simulink model "OpenLoop"  (R2022b)
settings: Solver=ode1  StartTime=0.0  StopTime=10  FixedStep=0.002  RelTol=1e-3  EnableMultiTasking=on
undefined symbols (not defined in the file or in its folder): sigbuilder_block
libraries: simulink x1
settings Model: SimulationMode=external  ExtModeTrigDuration=2  Creator=Alex  LastModifiedBy=lgoudal
settings SolverCC: AlgebraicLoopSolver=TrustRegion
settings DataIOCC: SaveFormat=StructureWithTime  ReturnWorkspaceOutputs=off
settings OptimizationCC: PassReuseOutputArgsAs=Individual arguments  MaxStackSize=64  EfficientTunableParamExpr=on
settings DebuggingCC: ParameterTunabilityLossMsg=error  UnconnectedInputMsg=warning  UnconnectedOutputMsg=warning  UnconnectedLineMsg=warning  SFMachineParentedDataDiag=warning  ArithmeticOperatorsInVariantConditions=warning
settings HardwareCC: ProdBitPerInt=16  ProdBitPerPointer=16  ProdBitPerSizeT=16  ProdBitPerPtrDiffT=16  ProdLargestAtomicFloat=None  ProdWordSize=8  ProdHWDeviceType=Atmel->AVR
settings ModelReferenceCC: EnableRefExpFcnMdlSchedulingChecks=on
settings SFSimCC: SimUseLocalCustomCode=off  MATLABDynamicMemAlloc=off  CustomCodeUndefinedFunction=UseInterfaceOnly
settings RTWCC: Description=Embedded Coder  SystemTargetFile=ert.tlc  HardwareBoard=Arduino Mega 2560  TemplateMakefile=ert_default_tmf  RTWUseLocalCustomCode=off  Toolchain=Arduino AVR  BuildConfiguration=Faster Runs  IncludeHyperlinkInReport=on  DLArmComputeVersion=19.05
settings CodeAppCC: ForceParamTrailComments=on  IgnoreCustomStorageClasses=off  OperatorAnnotations=on  SimulinkDataObjDesc=on  SFDataObjDesc=on  InsertBlockDesc=on
settings ERTTargetCC: SupportContinuousTime=on  SupportVariableSizeSignals=on  ExtMode=on  ExtModeTransport=3  ExtModeStaticAlloc=on  ExtModeMexFile=ext_xcp  ExtModeMexArgs=0 10 115200  ExtModeIntrfLevel=Level2 - Open

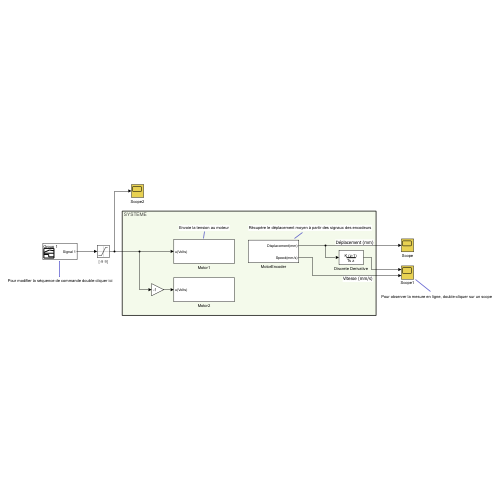
[thumbnail: Simulink's stored preview of the top-level diagram]
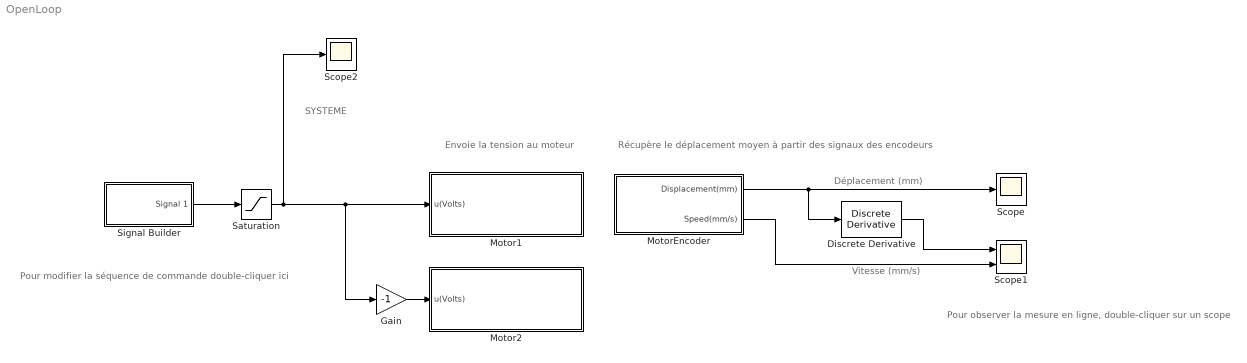
== system OpenLoop ==
  note: Déplacement (mm)
  note: Vitesse (mm/s)
  note: SYSTEME
  note: Récupère le déplacement moyen à partir des signaux des encodeurs
  note: Envoie la tension au moteur
  note: Pour observer la mesure en ligne, double-cliquer sur un scope
  note: Pour modifier la séquence de commande double-cliquer ici
  Discrete Derivative : simulink/Discrete/Discrete Derivative  gainval=1.0  ICPrevScaledInput=0.0  OutMin=[]  OutMax=[]  OutDataType=fixdt(1, 16)  OutScaling=2^-10  DoSatur=off
  Gain : Gain  Gain=-1
  Motor1 : Subsystem  mask{Vmax=12}
      mask prompts: Vmax "Power supply Voltage"
  Motor2 : Subsystem  mask{Vmax=12}
      mask prompts: Vmax "Power supply Voltage"
  MotorEncoder : Subsystem  mask{pulsePerTurn=8, beltPitch=2.032, nTeeth=90, gearRatio=46}
      mask prompts: pulsePerTurn "Encoder resolution"; beltPitch "Belt Pitch"; nTeeth "Number of teeth"; gearRatio "Gear ratio"
  Saturation : Saturate  UpperLimit=9  LowerLimit=-9
      settings: AttributesFormatString=[%<LowerLimit> %<UpperLimit>]
  Scope : Scope
  Scope1 : Scope  NumInputPorts=2
  Scope2 : Scope
  Signal Builder : Subsystem  Tag=STV Subsys  LoadFcn=sigbuilder_block('load');  StartFcn=sigbuilder_block('start');  StopFcn=sigbuilder_block('stop');  ClipboardFcn=sigbuilder_block('clipboard');  mask(Sigbuilder block){tuvar=[0:10]}
      mask help: Simulink:masks:SigbuilderBlock_MD
      mask init:
      | if ~strcmp(get_param(bdroot(gcbh),'SimulationStatus'),'stopped') tuvar = sigbuilder_block('maskInit'); end
      settings: CopyFcn=sigbuilder_block('copy');  DeleteFcn=sigbuilder_block('delete');  ModelCloseFcn=sigbuilder_block('modelClose');  PreSaveFcn=sigbuilder_block('preSave');  PauseFcn=sigbuilder_block('pause');  ContinueFcn=sigbuilder_block('continue');  NameChangeFcn=sigbuilder_block('namechange');  OpenFcn=sigbuilder_block('open',[382.125 217.125 550.5 400.5 ]);  CloseFcn=sigbuilder_block('close');
      mask Display: plot(0, 0, 100, 100,[2, 2, 32, 32, 2], [68, 8, 8, 68, 68],[32, 2], [38, 38], [32, 19, 2],[53, 60, 44], [32, 17, 17, 2],[16, 16, 31, 31]);txt = getActiveGroup(gcbh);text(2, 100, txt,'verticalAlignment', 'top');
  wires:
  MotorEncoder/1(Displacement(mm)) -> Scope/1, Discrete Derivative/1
  Signal Builder/1(Signal 1) -> Saturation/1
  Saturation/1 -> Gain/1, Motor1/1(u(Volts)), Scope2/1
  Discrete Derivative/1 -> Scope1/1
  MotorEncoder/2(Speed(mm/s)) -> Scope1/2
  Gain/1 -> Motor2/1(u(Volts))

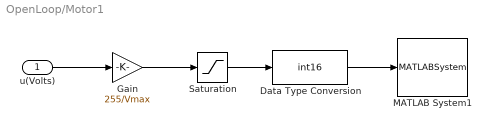
== system OpenLoop/Motor1 ==
  u(Volts) : Inport
  Data Type Conversion : DataTypeConversion  OutDataTypeStr=int16  SaturateOnIntegerOverflow=off  RndMeth=Floor
  Gain : Gain  Gain=255/Vmax
      settings: AttributesFormatString=%<Gain>
  MATLAB System1 : MATLABSystem  System=DCMotor1Set
      mask Type: DCMotor1Set
      mask Display:
      | disp('DC Motor 1');
      | port_label('input',1,'u');
  Saturation : Saturate  UpperLimit=255  LowerLimit=-255
  wires:
  Gain/1 -> Saturation/1
  u(Volts)/1 -> Gain/1
  Data Type Conversion/1 -> MATLAB System1/1
  Saturation/1 -> Data Type Conversion/1

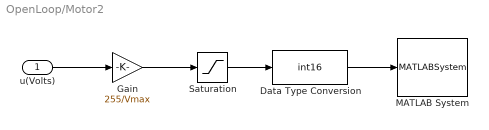
== system OpenLoop/Motor2 ==
  u(Volts) : Inport
  Data Type Conversion : DataTypeConversion  OutDataTypeStr=int16  SaturateOnIntegerOverflow=off  RndMeth=Floor
  Gain : Gain  Gain=255/Vmax
      settings: AttributesFormatString=%<Gain>
  MATLAB System : MATLABSystem  System=DCMotor2Set
      mask Type: DCMotor2Set
      mask Display:
      | disp('DC Motor 2');
      | port_label('input',1,'u');
  Saturation : Saturate  UpperLimit=255  LowerLimit=-255
  wires:
  Saturation/1 -> Data Type Conversion/1
  Data Type Conversion/1 -> MATLAB System/1
  u(Volts)/1 -> Gain/1
  Gain/1 -> Saturation/1

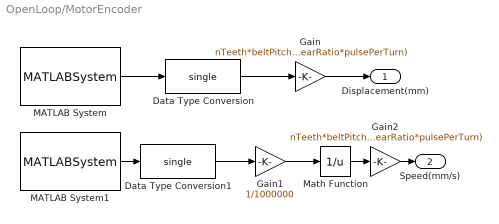
== system OpenLoop/MotorEncoder ==
  Data Type Conversion : DataTypeConversion  OutDataTypeStr=single  SaturateOnIntegerOverflow=off  RndMeth=Floor
  Data Type Conversion1 : DataTypeConversion  OutDataTypeStr=single  SaturateOnIntegerOverflow=off  RndMeth=Floor
  Gain : Gain  Gain=nTeeth*beltPitch/(gearRatio*pulsePerTurn)  OutDataTypeStr=single
      settings: AttributesFormatString=%<Gain>
  Gain1 : Gain  Gain=1/1000000
  Gain2 : Gain  Gain=nTeeth*beltPitch/(gearRatio*pulsePerTurn)  OutDataTypeStr=single
      settings: AttributesFormatString=%<Gain>
  MATLAB System : MATLABSystem  System=Enc1Read  SampleTime=0.002
      mask Type: Enc1Read
      mask Display:
      | disp('Encoder 1');
      | port_label('output',1,'y');
  MATLAB System1 : MATLABSystem  System=Enc1Period  SampleTime=0.002
      mask Type: Enc1Period
      mask Display:
      | disp('Encoder Period 1');
      | port_label('output',1,'y');
  Math Function : Math  Operator=reciprocal  SignedPower=on  OutputSignalType=real  OutDataTypeStr=single  SaturateOnIntegerOverflow=off
  Displacement(mm) : Outport  VectorParamsAs1DForOutWhenUnconnected=off
  Speed(mm/s) : Outport  Port=2  VectorParamsAs1DForOutWhenUnconnected=off
  wires:
  MATLAB System/1 -> Data Type Conversion/1
  Gain/1 -> Displacement(mm)/1
  Data Type Conversion/1 -> Gain/1
  Gain1/1 -> Math Function/1
  Data Type Conversion1/1 -> Gain1/1
  MATLAB System1/1 -> Data Type Conversion1/1
  Math Function/1 -> Gain2/1
  Gain2/1 -> Speed(mm/s)/1

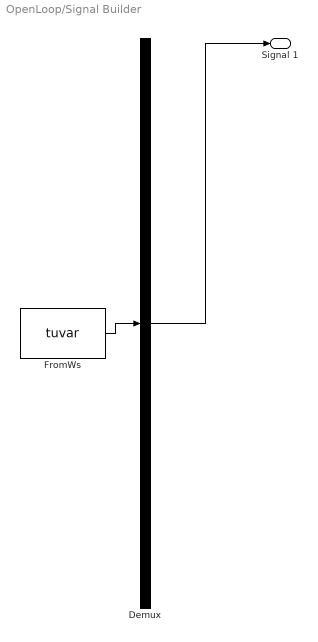
== system OpenLoop/Signal Builder ==
  Demux : Demux  Tag=STV Demux  Outputs=1
      settings: DisplayOption=none
  FromWs : FromWorkspace  Tag=STV FromWs  VariableName=tuvar
      SigBuilderData=|
      | common.afterFinalStr = 'Extrapolate'
      | common.sampleTime = 0
      | dataSet.timeRange = [0 10]
      | dataSet.name = 'Group 1'
      | sbobj.Groups.Name = 'Group 1'
      | sbobj.Groups.Signals.Name = 'Signal 1'
      | sbobj.Groups.Signals.XData = [0 1 1 1.5 1.5 4 4 5 5 7 7 8 8 9 9 9.5 9.5 10]
      | sbobj.Groups.Signals.YData = [0 0 7 7 0 0 4 4 0 0 -4 -4 0 0 -7 -7 0 0]
  Signal 1 : Outport  Tag=STV Outport  VectorParamsAs1DForOutWhenUnconnected=off
  wires:
  Demux/1 -> Signal 1/1
  FromWs/1 -> Demux/1
